simulink model "LQ_HW"  (R2023a)
settings: Solver=FixedStepAuto  StartTime=0.0  StopTime=inf  FixedStep=0.001  RelTol=1e-3  EnableMultiTasking=on
undefined symbols (not defined in the file): dev, klq, Main, pwm_output0, R
libraries: px4Sensorslib x2, px4lib x1
settings Model: SimulationMode=external  ExtModeTrigDuration=10  Creator=ArriGE66  LastModifiedBy=matte
settings SolverCC: PositivePriorityOrder=on
settings OptimizationCC: EnhancedBackFolding=on  PassReuseOutputArgsAs=Individual arguments  ZeroExternalMemoryAtStartup=off  ZeroInternalMemoryAtStartup=off  MaxStackSize=64  OptimizeBlockOrder=speed  DifferentSizesBufferReuse=on  EfficientTunableParamExpr=on
settings DebuggingCC: ParameterTunabilityLossMsg=error
settings HardwareCC: ProdBitPerPointer=32  ProdBitPerSizeT=32  ProdBitPerPtrDiffT=32  ProdLargestAtomicInteger=Long  ProdLargestAtomicFloat=Double  ProdWordSize=32  ProdLongLongMode=on  ProdHWDeviceType=ARM Compatible->ARM Cortex
settings SFSimCC: MATLABDynamicMemAlloc=off  SimTargetLang=C++
settings RTWCC: Description=Embedded Coder  SystemTargetFile=ert.tlc  HardwareBoard=PX4 Cube Orange  TemplateMakefile=ert_default_tmf  Toolchain=GNU Tools for PX4 Autopilots  TargetLang=C++
settings CodeAppCC: ForceParamTrailComments=on  IgnoreCustomStorageClasses=off  OperatorAnnotations=on  SimulinkDataObjDesc=on  SFDataObjDesc=on  InsertBlockDesc=on
settings ERTTargetCC: ExtMode=on  ExtModeTransport=3  ExtModeStaticAlloc=on  ExtModeStaticAllocSize=1024  ExtModeMexFile=ext_xcp  ExtModeMexArgs=1 COM10 3000000  ExtModeIntrfLevel=Level2 - Open

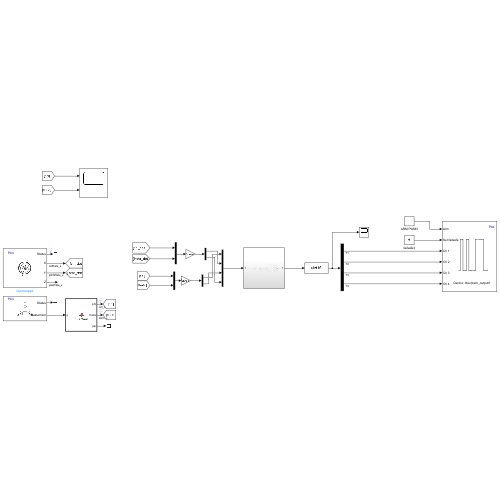
[thumbnail: Simulink's stored preview of the top-level diagram]
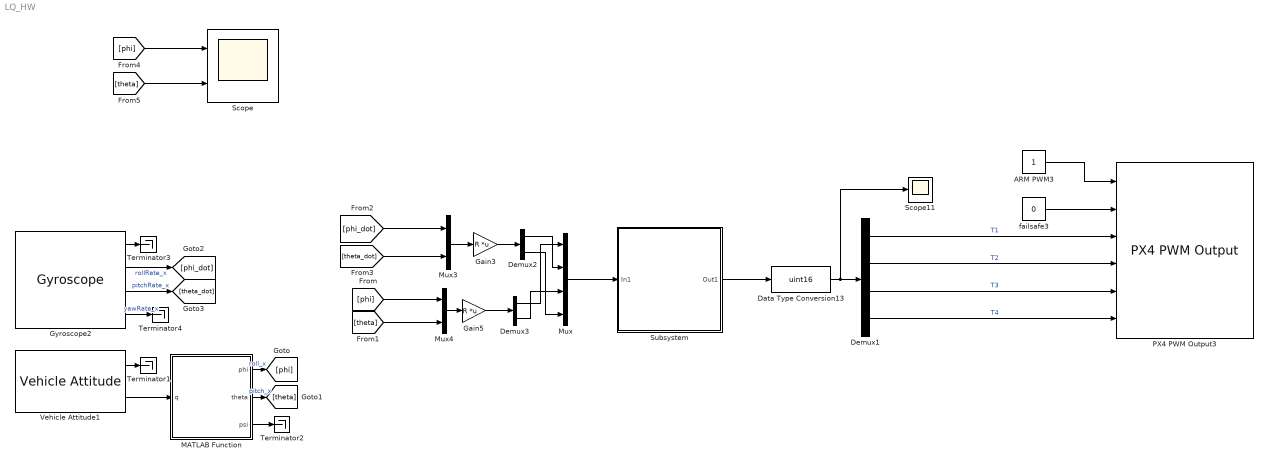
== system LQ_HW ==
  ARM PWM3 : Constant  OutDataTypeStr=boolean  SampleTime=0.002
  Data Type Conversion13 : DataTypeConversion  OutDataTypeStr=uint16  SaturateOnIntegerOverflow=off  RndMeth=Floor
  Demux1 : Demux
  Demux2 : Demux  Outputs=2
  Demux3 : Demux  Outputs=2
  Gain3 : Gain  Gain=R  Multiplication=Matrix(K*u) (u vector)
  Gain5 : Gain  Gain=R  Multiplication=Matrix(K*u) (u vector)
  Gyroscope2 : px4Sensorslib/Gyroscope  uorbTimeStamp=off  BlockingMode=off  BlockTimeout=1e-3  sampleTime=0.002
  MATLAB Function : MATLAB Function  TreatAsAtomicUnit=on
  Mux : Mux
  Mux3 : Mux  Inputs=2
  Mux4 : Mux  Inputs=2
  PX4 PWM Output3 : px4lib/PX4 PWM Output  pwmDevice=Main (/dev/pwm_output0)  pwmChannel1_=on  pwmChannel2_=on  pwmChannel3_=on  pwmChannel4_=on  pwmChannel5_=off  pwmChannel6_=off  pwmChannel7_=off  pwmChannel8_=off  forceTerminateFailsafe=off  outputErrorStatus=off
  Scope : Scope  NumInputPorts=2
  Scope11 : Scope
  Subsystem : Subsystem
  Terminator{1..4} (4 alike) : Terminator
  Vehicle Attitude1 : px4Sensorslib/Vehicle Attitude  rollRate=off  pitchRate=off  yawRate=off  quaternion=on  uorbTimeStamp=off  BlockingMode=off  BlockTimeout=0.001  sampleTime=0.002
  failsafe3 : Constant  Value=0  OutDataTypeStr=boolean  SampleTime=0.002
  wires:
  Data Type Conversion13/1 -> Scope11/1, Demux1/1
  Demux1/1 -> PX4 PWM Output3/3  "T1"
  Demux1/2 -> PX4 PWM Output3/4  "T2"
  ARM PWM3/1 -> PX4 PWM Output3/1
  failsafe3/1 -> PX4 PWM Output3/2
  Vehicle Attitude1/2 -> MATLAB Function/1(q)
  MATLAB Function/3(psi) -> Terminator2/1
  Demux1/3 -> PX4 PWM Output3/5  "T3"
  Demux1/4 -> PX4 PWM Output3/6  "T4"
  Vehicle Attitude1/1 -> Terminator1/1
  Gyroscope2/1 -> Terminator3/1
  Mux3/1 -> Gain3/1
  Gain3/1 -> Demux2/1
  Mux4/1 -> Gain5/1
  Gain5/1 -> Demux3/1
  Demux2/1 -> Mux/2
  Demux3/1 -> Mux/1
  Demux3/2 -> Mux/3
  Demux2/2 -> Mux/4
  Mux/1 -> Subsystem/1(In1)
  Subsystem/1(Out1) -> Data Type Conversion13/1
  MATLAB Function/1(phi) -> [phi]  "roll_x"
  MATLAB Function/2(theta) -> [theta]  "pitch_x"
  [phi] -> Mux4/1
  [theta] -> Mux4/2
  Gyroscope2/2 -> [phi_dot]  "rollRate_x"
  Gyroscope2/3 -> [theta_dot]  "pitchRate_x"
  Gyroscope2/4 -> Terminator4/1  "yawRate_x"
  [phi_dot] -> Mux3/1
  [theta_dot] -> Mux3/2
  [phi] -> Scope/1
  [theta] -> Scope/2

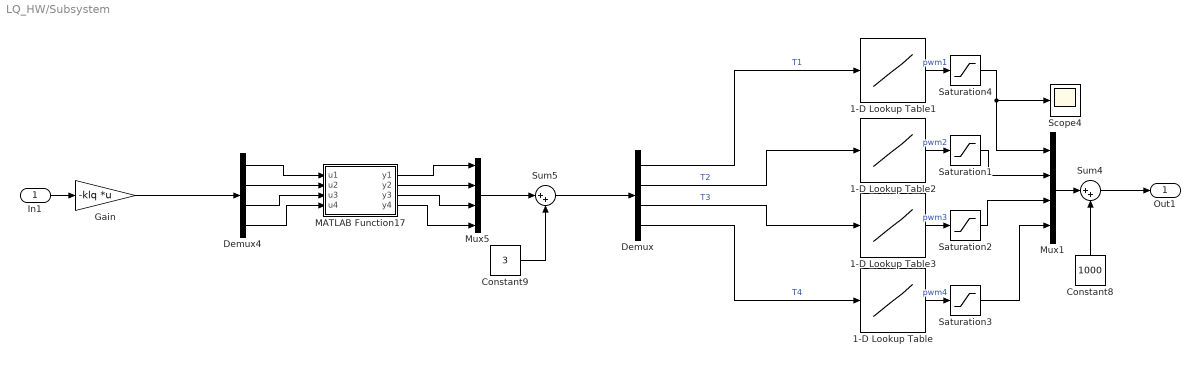
== system LQ_HW/Subsystem ==
  In1 : Inport
  1-D Lookup Table : Lookup_n-D  NumberOfTableDimensions=1  BreakpointsForDimension1=[0;0.06477642396;0.16;0.63;2.44;4.43;6.92;8.77;10.52;11.63;12.03;12.09;12.091;12.092;12.093;12.094;12.095;12.096;12.097;12.098;12.099]  Table=[0;50;100;150;200;250;300;350;400;450;500;550;600;650;700;750;800;850;900;950;1000]  InternalRulePriority=Speed  RndMeth=Simplest
  1-D Lookup Table1 : Lookup_n-D  NumberOfTableDimensions=1  BreakpointsForDimension1=[0;0.02;0.06;0.29;0.73;1.07;1.88;2.91;4;5.06;6.71;7.86;9.41;10.86;11.45;11.82;12.07;12.31;12.52;12.74;12.75]  Table=[0;50;100;150;200;250;300;350;400;450;500;550;600;650;700;750;800;850;900;950;1000]  InternalRulePriority=Speed  RndMeth=Simplest
  1-D Lookup Table2 : Lookup_n-D  NumberOfTableDimensions=1  BreakpointsForDimension1=[0;0.05;0.39;1.67;3.19;5.57;8.07;10.01;10.71;11.06;11.42;11.53;11.55;11.551;11.552;11.553;11.554;11.555;11.556;11.557;11.558]  Table=[0;50;100;150;200;250;300;350;400;450;500;550;600;650;700;750;800;850;900;950;1000]  InternalRulePriority=Speed  RndMeth=Simplest
  1-D Lookup Table3 : Lookup_n-D  NumberOfTableDimensions=1  BreakpointsForDimension1=[0;0.06;0.23;0.89;2.47;3.9;5.86;7.81;9.42;10.12;10.6;11.01;11.34;11.39;11.391;11.392;11.393;11.394;11.395;11.396;11.397]  Table=[0;50;100;150;200;250;300;350;400;450;500;550;600;650;700;750;800;850;900;950;1000]  InternalRulePriority=Speed  RndMeth=Simplest
  Constant8 : Constant  Value=1000
  Constant9 : Constant  Value=3
  Demux : Demux
  Demux4 : Demux
  Gain : Gain  Gain=-klq  Multiplication=Matrix(K*u) (u vector)
  MATLAB Function17 : MATLAB Function  TreatAsAtomicUnit=on
  Mux1 : Mux
  Mux5 : Mux
  Saturation{1..4} (4 alike) : Saturate  UpperLimit=1000  LowerLimit=0
  Scope4 : Scope
  Sum4 : Sum  Inputs=|++
  Sum5 : Sum  Inputs=|++
  Out1 : Outport
  wires:
  1-D Lookup Table/1 -> Saturation3/1  "pwm4"
  1-D Lookup Table3/1 -> Saturation2/1  "pwm3"
  Demux/1 -> 1-D Lookup Table1/1  "T1"
  Saturation4/1 -> Scope4/1, Mux1/1
  Mux1/1 -> Sum4/1
  Saturation3/1 -> Mux1/4
  1-D Lookup Table2/1 -> Saturation1/1  "pwm2"
  1-D Lookup Table1/1 -> Saturation4/1  "pwm1"
  In1/1 -> Gain/1
  Saturation2/1 -> Mux1/3
  Saturation1/1 -> Mux1/2
  Constant8/1 -> Sum4/2
  Demux4/2 -> MATLAB Function17/2(u2)
  Sum5/1 -> Demux/1
  Demux/2 -> 1-D Lookup Table2/1  "T2"
  Demux4/1 -> MATLAB Function17/1(u1)
  Sum4/1 -> Out1/1
  Demux/4 -> 1-D Lookup Table/1  "T4"
  Demux/3 -> 1-D Lookup Table3/1  "T3"
  MATLAB Function17/2(y2) -> Mux5/2
  MATLAB Function17/4(y4) -> Mux5/4
  Demux4/3 -> MATLAB Function17/3(u3)
  MATLAB Function17/1(y1) -> Mux5/1
  Demux4/4 -> MATLAB Function17/4(u4)
  MATLAB Function17/3(y3) -> Mux5/3
  Mux5/1 -> Sum5/1
  Gain/1 -> Demux4/1
  Constant9/1 -> Sum5/2

== matlab function LQ_HW/MATLAB Function ==
  data: q input; phi output; theta output; psi output
function [phi,theta,psi] = quat2eul(q)
% Conversion from Quaternion to Euler angles based on the PX4 Firmware
% v1.6.5 release.
% 
% Quaternion -> DCM -> Euler Angles
% INPUT:
%   q: Quaternion vector of the format: (a + bi + cj + dk)
% OUTPUT:
%   [phi,theta,psi]: Euler angles in radians.
% 
 
    a = q(1);
    b = q(2);
    c = q(3);
    d = q(4);

    aSq = a*a;
    bSq = b*b;
    cSq = c*c;
    dSq = d*d;

    d_pi2 = pi/2;

    % quaternion_to_dcm
    dcm00 = aSq + bSq - cSq - dSq;
    % dcm01 = 2*(b*c - a*d);
    dcm02 = 2*(a*c + b*d);
    dcm10 = 2*(b*c + a*d);
    % dcm11 = aSq - bSq + cSq - dSq;
    dcm12 = 2*(c*d - a*b);
    dcm20 = 2*(b*d - a*c);
    dcm21 = 2*(a*b + c*d);
    dcm22 = aSq - bSq - cSq + dSq;

    % dcm_to_euler
    theta = asin(-dcm20);
    if abs(theta - d_pi2) < 1.0e-3
        phi = single(0.0);
        psi = atan2(dcm12, dcm02);
    elseif abs(theta + d_pi2) < 1.0e-3
        phi = single(0.0);
        psi = atan2(-dcm12, -dcm02);
    else
        phi = atan2(dcm21, dcm22);
        psi = atan2(dcm10, dcm00);
    end

end

== matlab function LQ_HW/Subsystem/MATLAB Function17 ==
  data: u1 input; y1 output; u2 input; u3 input; u4 input; y2 output; y3 output; y4 output
function [y1,y2,y3,y4] = fcn(u1,u2,u3,u4)

if u1 < 0
    u2 = u2 + abs(u1);
    u1 = u1+abs(u1);
end
if u2 < 0
    u2 = u2 + abs(u2);
    u1 = u1 + abs(u2);
end
if u3 < 0
    u3 = u3 + abs(u3);
    u4 = u4 + abs(u3);
end    
if u4 < 0
    u4 = u4 + abs(u4);
    u3 = u3 + abs(u4);
end
 y1 = u1;
 y2 = u2;
 y3 = u3;
 y4 = u4;
